simulink model "testChild"  (R2023b)
settings: Solver=VariableStepAuto  StartTime=0.0  StopTime=10.0  RelTol=1e-3
model workspace (MAT data in the model file):
  s = Simulink.Parameter
  s.Value.a = 2
  s.Value.b = 3
  s.DataType = 'Bus: slBus1'
  s.Complexity = 'real'
  s.Dimensions = [1 1]
values from neighbouring files (symbols this model uses):
  s = 2.0    [busesDD.sldd]
settings Model: DataDictionary=busesDD.sldd  ParameterArgumentNames=s  Creator=grouleau  LastModifiedBy=grouleau

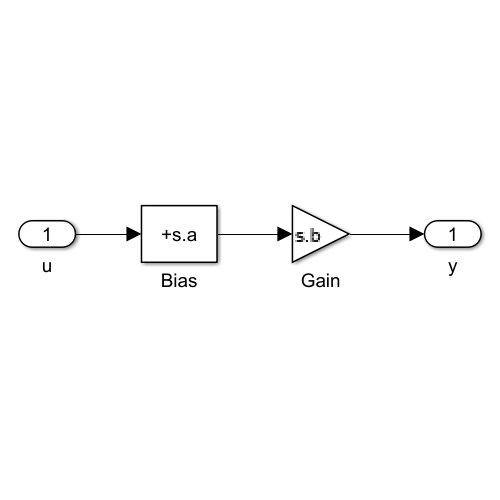
[thumbnail: Simulink's stored preview of the top-level diagram]
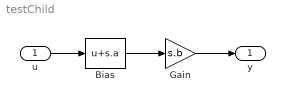
== system testChild ==
  u : Inport
  Bias : Bias  Bias=s.a  SaturateOnIntegerOverflow=off
  Gain : Gain  Gain=s.b
  y : Outport
  wires:
  u/1 -> Bias/1
  Gain/1 -> y/1
  Bias/1 -> Gain/1
